simulink model "fangzhen1"  (R2014a)
settings: Solver=ode45  StartTime=0.0  StopTime=0.5  RelTol=1e-3
settings Model: Creator=HZQ  LastModifiedBy=HZQ

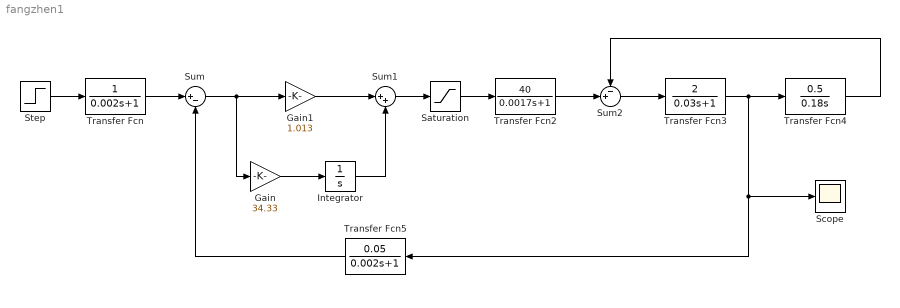
== system fangzhen1 ==
  Gain : Gain  Gain=34.33
  Gain1 : Gain  Gain=1.013
  Integrator : Integrator
  Saturation : Saturate  UpperLimit=10  LowerLimit=-10
  Scope : Scope
      settings: TimeRange=2
  Step : Step  Before=10  After=0  SampleTime=0
  Sum : Sum  Inputs=|+-
  Sum1 : Sum  Inputs=|++
  Sum2 : Sum  Inputs=-+|
  Transfer Fcn : TransferFcn  Denominator=[0.002 1]
  Transfer Fcn2 : TransferFcn  Numerator=[40]  Denominator=[0.0017 1]
  Transfer Fcn3 : TransferFcn  Numerator=[2]  Denominator=[0.03 1]
  Transfer Fcn4 : TransferFcn  Numerator=[0.5]  Denominator=[0.18 0]
  Transfer Fcn5 : TransferFcn  Numerator=[0.05]  Denominator=[0.002 1]
  wires:
  Step/1 -> Transfer Fcn/1
  Transfer Fcn/1 -> Sum/1
  Sum/1 -> Gain1/1, Gain/1
  Gain/1 -> Integrator/1
  Gain1/1 -> Sum1/1
  Integrator/1 -> Sum1/2
  Transfer Fcn2/1 -> Sum2/2
  Sum2/1 -> Transfer Fcn3/1
  Sum1/1 -> Saturation/1
  Saturation/1 -> Transfer Fcn2/1
  Transfer Fcn3/1 -> Scope/1, Transfer Fcn5/1, Transfer Fcn4/1
  Transfer Fcn4/1 -> Sum2/1
  Transfer Fcn5/1 -> Sum/2
